simulink model "Digital_manipulation"  (R2021a)
settings: Solver=VariableStepAuto  StartTime=0.0  StopTime=1  MaxStep=1e-5  RelTol=1e-3
libraries: dspfdesign x2, commdigbbndpm3 x2, commsink2 x1, commrandsrc3 x1, commchan3 x1
settings Model: Creator=Gleb  LastModifiedBy=Gleb
settings SolverCC: AlgebraicLoopSolver=TrustRegion
settings DebuggingCC: SFMachineParentedDataDiag=warning

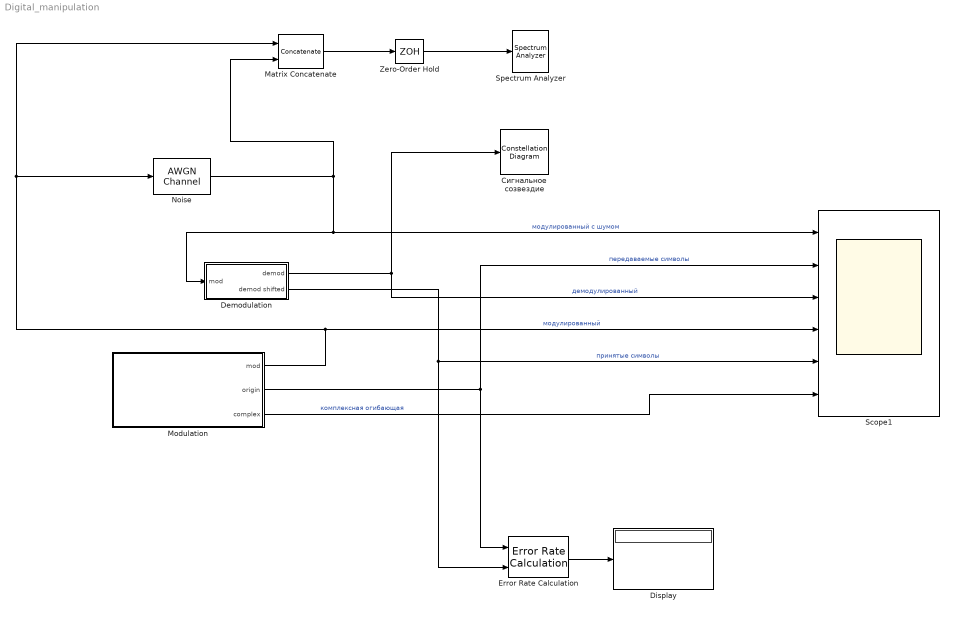
== system Digital_manipulation ==
  Demodulation : Subsystem  mask{SamplingFrequency=1e5, Uc=1e4, SymbolRate=1e3}
      mask prompts: SamplingFrequency "Частота дискретизации, Гц"; Uc "Частота несущей, Гц"; SymbolRate "Символьная скорость, сим/сек"
  Display : Display
  Error Rate Calculation : commsink2/Error Rate Calculation  N=1  st_delay=0  cp_mode=Entire frame  subframe=[]  PMode=Port  WsName=BER  RsMode2=off  stop=off  numErr=100  maxBits=1e6
  Matrix Concatenate : Concatenate  Mode=Multidimensional array  ConcatenateDimension=2
  Modulation : Subsystem  mask{Uc=1e4, SymbolRate=1e3, SamplingFrequency=1e5}
      mask prompts: Uc "Несущая частота, Гц"; SymbolRate "Символьная скорость, сим/сек"; SamplingFrequency "Частота дискретизации, Гц"
  Noise : commchan3/AWGN Channel  InputProcessing=Columns as channels (frame based)  seed=67  noiseMode="Signal to noise ratio  (SNR)"  EbNodB=20  EsNodB=10  SNRdB=5  bitsPerSym=2  Ps=1  Tsym=1/1000  variance=1
  Scope1 : Scope  NumInputPorts=6
  Spectrum Analyzer : SpectrumAnalyzer
  Zero-Order Hold : ZeroOrderHold  SampleTime=-1
  Сигнальное созвездие : ConstellationDiagram
  wires:
  Modulation/1(mod) -> Noise/1, Matrix Concatenate/1, Scope1/4  "модулированный"
  Modulation/2(origin) -> Scope1/2, Error Rate Calculation/1  "передаваемые символы"
  Noise/1 -> Scope1/1, Demodulation/1(mod), Matrix Concatenate/2  "модулированный с шумом"
  Modulation/3(complex) -> Scope1/6  "комплексная огибающая"
  Demodulation/2(demod shifted) -> Error Rate Calculation/2, Scope1/5  "принятые символы"
  Demodulation/1(demod) -> Scope1/3, Сигнальное созвездие/1  "демодулированный"
  Matrix Concatenate/1 -> Zero-Order Hold/1
  Zero-Order Hold/1 -> Spectrum Analyzer/1
  Error Rate Calculation/1 -> Display/1

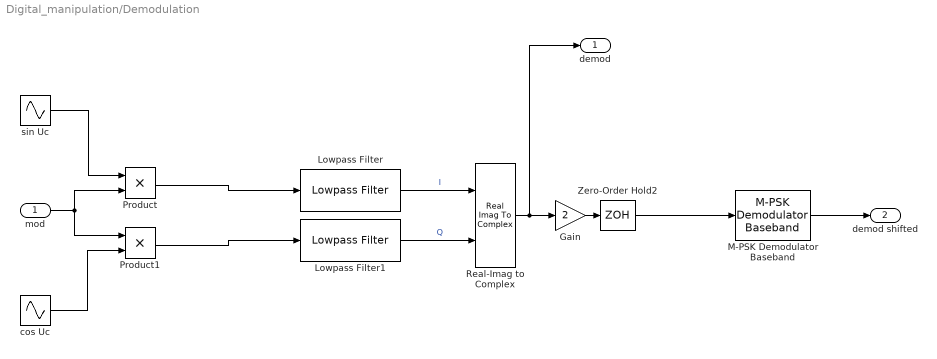
== system Digital_manipulation/Demodulation ==
  mod : Inport
  Gain : Gain  Gain=2
  Lowpass Filter : dspfdesign/Lowpass Filter  FilterType=FIR  DesignForMinimumOrder=on  FilterOrder=50  PassbandFrequency=Uc  StopbandFrequency=1.2*Uc  PassbandRipple=0.5  StopbandAttenuation=80  InheritSampleRate=off  SampleRate=SamplingFrequency  SimulateUsing=Interpreted execution  roundingMode=Floor  coeffsDataTypeStr=fixdt(1,16)
  Lowpass Filter1 : dspfdesign/Lowpass Filter  FilterType=FIR  DesignForMinimumOrder=on  FilterOrder=50  PassbandFrequency=Uc  StopbandFrequency=1.2*Uc  PassbandRipple=0.5  StopbandAttenuation=80  InheritSampleRate=off  SampleRate=SamplingFrequency  SimulateUsing=Interpreted execution  roundingMode=Floor  coeffsDataTypeStr=fixdt(1,16)
  M-PSK Demodulator Baseband : commdigbbndpm3/M-PSK Demodulator Baseband  M=4  OutType=Integer  DecType=Hard decision  VarSource=Dialog  Variance=1  Dec=Gray  Mapping=[0:7]  Ph=pi/4  outDtype1=Inherit via internal rule  outDtype2=Inherit via internal rule  derotateFactorWordLen=16  derotateFactorDataTypeStr=Inherit: Same word length as input  derotateFactorLastDataTypeStr=Inherit: Same word length as input
  Product : Product
  Product1 : Product
  Real-Imag to Complex : RealImagToComplex
  Zero-Order Hold2 : ZeroOrderHold  SampleTime=1/SymbolRate
  cos Uc : Sin  Frequency=2*pi*Uc  Phase=pi/2  SampleTime=1/SamplingFrequency
  sin Uc : Sin  Frequency=2*pi*Uc  SampleTime=1/SamplingFrequency
  demod : Outport
  demod shifted : Outport  Port=2
  wires:
  mod/1 -> Product1/1, Product/2
  sin Uc/1 -> Product/1
  Product/1 -> Lowpass Filter/1
  cos Uc/1 -> Product1/2
  Product1/1 -> Lowpass Filter1/1
  Lowpass Filter1/1 -> Real-Imag to Complex/2  "Q"
  Lowpass Filter/1 -> Real-Imag to Complex/1  "I"
  Real-Imag to Complex/1 -> demod/1, Gain/1
  M-PSK Demodulator Baseband/1 -> demod shifted/1
  Gain/1 -> Zero-Order Hold2/1
  Zero-Order Hold2/1 -> M-PSK Demodulator Baseband/1

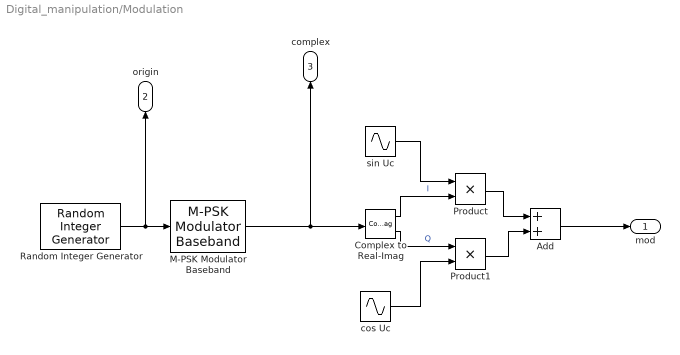
== system Digital_manipulation/Modulation ==
  Add : Sum
  Complex to Real-Imag : ComplexToRealImag
  M-PSK Modulator Baseband : commdigbbndpm3/M-PSK Modulator Baseband  M=4  InType=Integer  Enc=Gray  Mapping=[0:7]  Ph=pi/4  outDtype=double  outWordLen=16  outUDDataType=sfix(16)  outFracLenMode=Best precision  outFracLen=15  outDataTypeStr=double  outLastDataTypeStr=double
  Product : Product
  Product1 : Product
  Random Integer Generator : commrandsrc3/Random Integer Generator  SetSize=4  SeedSource=Auto  Seed=0  SampleTime=1/SymbolRate  SamplesPerFrame=1  OutputDataType=uint8  SimulateUsing=Interpreted execution
  cos Uc : Sin  Frequency=2*pi*Uc  Phase=pi/2  SampleTime=1/SamplingFrequency
  sin Uc : Sin  Frequency=2*pi*Uc  SampleTime=1/SamplingFrequency
  mod : Outport
  origin : Outport  Port=2
  complex : Outport  Port=3
  wires:
  cos Uc/1 -> Product1/2
  Complex to Real-Imag/1 -> Product/2  "I"
  sin Uc/1 -> Product/1
  Add/1 -> mod/1
  Random Integer Generator/1 -> M-PSK Modulator Baseband/1, origin/1
  Product1/1 -> Add/2
  M-PSK Modulator Baseband/1 -> Complex to Real-Imag/1, complex/1
  Complex to Real-Imag/2 -> Product1/1  "Q"
  Product/1 -> Add/1
